simulink model "DC_Motor_PID_Control"  (R2024a)
settings: Solver=VariableStepAuto  StartTime=0.0  StopTime=10.0  RelTol=1e-3
libraries: spsControlledVoltageSourceLib x1, spsCurrentMeasurementLib x1, spsDCMachineLib x1, spsDCVoltageSourceLib x1, slpidlib x1, spspowerguiLib x1
settings Model: Creator=Anjali Sharma  LastModifiedBy=Anjali Sharma

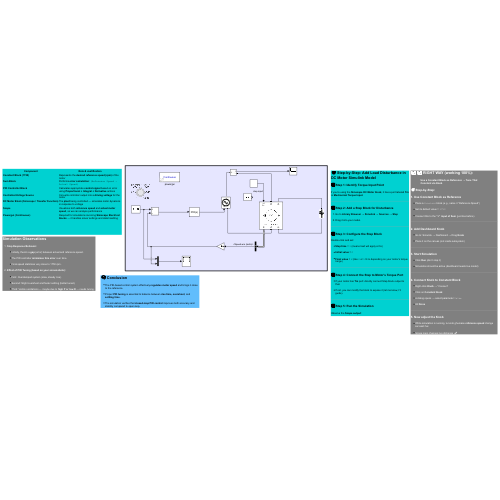
[thumbnail: Simulink's stored preview of the top-level diagram]
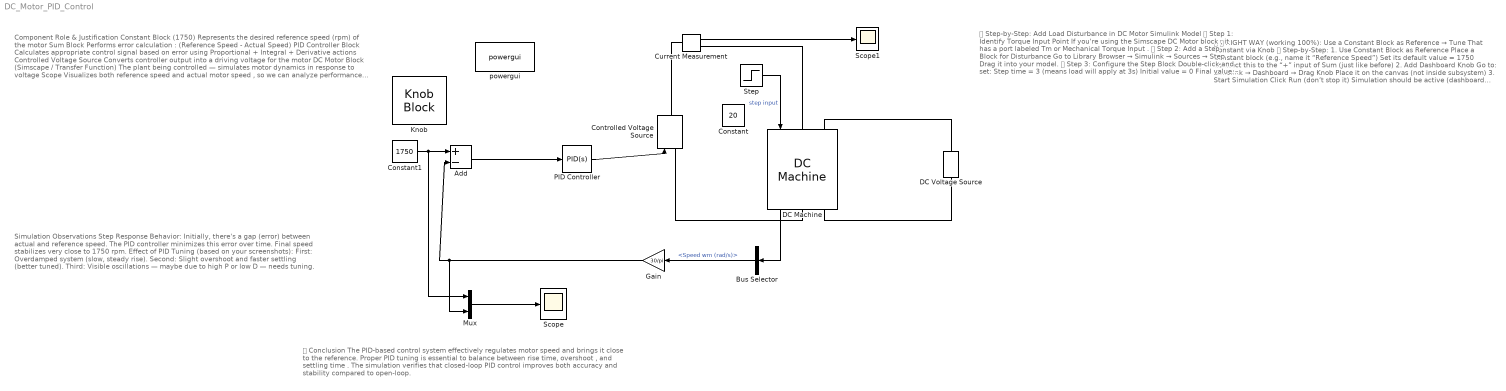
== system DC_Motor_PID_Control ==
  note: ✅ ✅ RIGHT WAY (working 100%):
      | Use a Constant Block as Reference → Tune That Constant via Knob
      | 🧭 Step-by-Step:
      | 1. Use Constant Block as Reference
      | Place a Constant block (e.g., name it “Reference Speed”)
      | Set its default value = 1750
      | Connect this to the “+” input of Sum (just like before)
      | 2. Add Dashboard Knob
      | Go to: Simulink → Dashboard → Drag Knob
      | Place it on the canvas (not inside subsystem)
      | 3. Start Simulation
      | Click Run (don’t stop it)
      | Simulation should be active (dashboard needs live model)
      | 4. Connect Knob to Constant Block
      | Right-click Knob → “Connect”
      | Click on Constant block
      | A dialog opens → select parameter Value
      | Hit Done
      | 5. Now adjust the Knob
      | While simulation is running, tu knob ghumake reference speed change kar sakti hai
      | Scope mein changes live dikhenge 🚀
      | 🧪 Why PID can't directly accept knob:
      | Because the PID input is a dynamic signal , knob can only connect to tunable parameters (like value of Constant or Gain blocks) — not to arbitrary wires or results.
  note: 🧭 Step-by-Step: Add Load Disturbance in DC Motor Simulink Model
      | ✅ Step 1: Identify Torque Input Point
      | If you're using the Simscape DC Motor block , it has a port labeled Tm or Mechanical Torque Input .
      | ✅ Step 2: Add a Step Block for Disturbance
      | Go to Library Browser → Simulink → Sources → Step
      | Drag it into your model.
      | ✅ Step 3: Configure the Step Block
      | Double-click and set:
      | Step time = 3 (means load will apply at 3s)
      | Initial value = 0
      | Final value = X (like 2 or 5 N·m depending on your motor’s torque range)
      | ✅ Step 4: Connect the Step to Motor's Torque Port
      | If your motor has Tm port: directly connect Step block output to that.
      | If not, you can modify the block to expose it (let me know, I’ll guide).
      | ✅ Step 5: Run the Simulation
      | Observe the Scope output :
      | You’ll see a dip in speed at t = 3s due to load.
      | If PID is well-tuned, the motor should recover to 1750 rpm soon after.
      | 🎯 Bonus Tip:
      | Want to test PID strength ? Try:
      | Disturbance = 10 N·m (large)
      | Remove D term from PID → You'll see slower recovery or instability
  note: 🧠 Conclusion
      | The PID-based control system effectively regulates motor speed and brings it close to the reference.
      | Proper PID tuning is essential to balance between rise time, overshoot , and settling time .
      | The simulation verifies that closed-loop PID control improves both accuracy and stability compared to open-loop.
  note: Simulation Observations
      | Step Response Behavior: Initially, there's a gap (error) between actual and reference speed.
      | The PID controller minimizes this error over time.
      | Final speed stabilizes very close to 1750 rpm.
      |
      | Effect of PID Tuning (based on your screenshots): First: Overdamped system (slow, steady rise).
      | Second: Slight overshoot and faster settling (better tuned).
      | Third: Visible oscillations — maybe due to high P or low D — needs tuning.
  note: Component
      | Role & Justification
      |
      | Constant Block (1750)
      | Represents the desired reference speed (rpm) of the motor
      |
      | Sum Block
      | Performs error calculation : (Reference Speed - Actual Speed)
      |
      | PID Controller Block
      | Calculates appropriate control signal based on error using Proportional + Integral + Derivative actions
      |
      | Controlled Voltage Source
      | Converts controller output into a driving voltage for the motor
      |
      | DC Motor Block (Simscape / Transfer Function)
      | The plant being controlled — simulates motor dynamics in response to voltage
      |
      | Scope
      | Visualizes both reference speed and actual motor speed , so we can analyze performance
      |
      | Powergui (Continuous)
      | Required for simulations involving Simscape Electrical blocks — it handles solver settings and data handling
  Add : Sum  Inputs=+-
  Bus Selector : BusSelector  OutputSignals=Speed wm (rad/s)
  Constant : Constant  Value=20
  Constant1 : Constant  Value=1750
  Controlled Voltage Source : spsControlledVoltageSourceLib/Controlled Voltage Source  Initialize=on  Source_Type=AC  Amplitude=0  Phase=0  Frequency=0  Measurements=None
  Current Measurement : spsCurrentMeasurementLib/Current Measurement  PhasorSimulation=off  OutputType=Complex  PSBequivalent=0
  DC Machine : spsDCMachineLib/DC Machine  PresetModel=02: 5HP 240V 1750RPM Field:150V  MechanicalLoad=Torque TL  FieldType=Wound  ShowDetailedParameters=on  MeasurementBus=off  RLa=[0.78 0.016]  RLf=[150 112.5]  Laf=1.234  MachineConstant=Torque constant (N.m/A)  Ke=1.8  Kt=1.8  J=0.05  Bm=0.01  Tf=0  w0=1  Ifinit=1  TsPowergui=0  TsBlock=-1
  DC Voltage Source : spsDCVoltageSourceLib/DC Voltage Source  Amplitude=150  Measurements=None
  Gain : Gain  Gain=30/pi
  Knob : KnobBlock  ScaleMax=3000
  Mux : Mux  Inputs=2
  PID Controller : slpidlib/PID Controller  Controller=PID  Form=Parallel  TimeDomain=Continuous-time  UseExternalTs=off  SampleTime=-1  IntegratorMethod=Forward Euler  FilterMethod=Forward Euler  ControllerParametersSource=internal  P=0.214596036046498  I=5.26646706519129  UseKiTs=off  D=0.00216589040036506  UseExternalDerivativeSource=off  N=5488.43681333471  UseFilter=on  TunerSelectOption=Transfer Function Based (PID Tuner App)  InitialConditionSource=internal  InitialConditionForIntegrator=0  InitialConditionForFilter=0  DifferentiatorICPrevScaledInput=0  ExternalReset=none  TrackingMode=off  Kt=1  LimitOutput=off  SatLimitsSource=internal  UpperSaturationLimit=inf  LowerSaturationLimit=-inf  LinearizeAsGain=on  AntiWindupMode=none  Kb=1  LimitIntegrator=off  UpperIntegratorSaturationLimit=inf  LowerIntegratorSaturationLimit=-inf  POutMin=[]  POutMax=[]  IOutMin=[]  IOutMax=[]  DOutMin=[]  DOutMax=[]  NOutMin=[]  NOutMax=[]  SumOutMin=[]  SumOutMax=[]  SaturationOutMin=[]  SaturationOutMax=[]  PParamMin=[]  PParamMax=[]  IParamMin=[]  IParamMax=[]  DParamMin=[]  DParamMax=[]  NParamMin=[]  NParamMax=[]  KbParamMin=[]  KbParamMax=[]  KtParamMin=[]  KtParamMax=[]  KbOutMin=[]  KbOutMax=[]  KtOutMin=[]  KtOutMax=[]  IntegratorOutMin=[]  IntegratorOutMax=[]  FilterOutMin=[]  FilterOutMax=[]  SumI1OutMin=[]  SumI1OutMax=[]  SumI2OutMin=[]  SumI2OutMax=[]  SumI3OutMin=[]  SumI3OutMax=[]  SumI4OutMin=[]  SumI4OutMax=[]  SumDOutMin=[]  SumDOutMax=[]  DifferentiatorOutMin=[]  DifferentiatorOutMax=[]  FilterDiffOutCoefMin=[]  FilterDiffOutCoefMax=[]  ReciprocalOutMin=[]  ReciprocalOutMax=[]  SumDenOutMin=[]  SumDenOutMax=[]  SumNumOutMin=[]  SumNumOutMax=[]  DivideOutMin=[]  DivideOutMax=[]  UdiffTsProdOutMin=[]  UdiffTsProdOutMax=[]  NTsProdOutMin=[]  NTsProdOutMax=[]  UintegralTsProdOutMin=[]  UintegralTsProdOutMax=[]  UngainTsProdOutMin=[]  UngainTsProdOutMax=[]  ClampingZeroOutDataTypeStr=Inherit: Inherit via back propagation  ClampingZeroOutMin=[]  ClampingZeroOutMax=[]  FilterDenConstantOutDataTypeStr=Inherit: Inherit via back propagation  FilterDenConstantOutMin=[]  FilterDenConstantOutMax=[]  PCopyOutDataTypeStr=Inherit: Inherit via back propagation  PCopyOutMin=[]  PCopyOutMax=[]  NCopyOutDataTypeStr=Inherit: Inherit via back propagation  NCopyOutMin=[]  NCopyOutMax=[]  IntegratorContinuousStateAttributes=''  IntegratorStateMustResolveToSignalObject=off  IntegratorRTWStateStorageClass=Auto  FilterContinuousStateAttributes=''  FilterStateMustResolveToSignalObject=off  FilterRTWStateStorageClass=Auto  ParallelPVariant=InternalParameters  IdealPVariant=Disabled  IVariant=InternalParameters  DVariant=InternalParameters  IntegratorVariant=Continuous  SatVariant=Disabled  AWVariant=Passthrough  PCopyVariant=Disabled  TRVariant=Disabled  FdbkBlocksVariant=Forward  IdealPFdbkVariant=Disabled  SatFdbkVariant=Disabled  DerivativeFilterVariant=ContFilter  NVariant=InternalParameters  NCopyVariant=Disabled  FilterICVariant=InternalICsFilter  IntegratorICVariant=InternalICs  ExternalResetVariant=Disabled  TRSumVariant=Passthrough  SumFdbkVariant=Disabled  SumVariant=Sum_PID  TsampFilterVariant=InternalTs  TsampNgainVariant=Passthrough  TsampIntegralVariant=Disabled_SignalSpec  ExternalSaturationOutDataTypeStr=Inherit: Same as second input  DerivativeSourceVariant=ErrorSignal
  Scope : Scope
  Scope1 : Scope
  Step : Step  Time=3  After=2  SampleTime=0
  powergui : spspowerguiLib/powergui  Priority=1  SimulationMode=Continuous  SampleTime=50e-6  frequency=60  Iterations=50  frequencyindice=0  Pbase=100e6  ErrMax=1e-4  UnitsV=kV  UnitsW=MW  buscounter=0  FunctionMessages=off  echomessages=off  EnableUseOfTLC=off  CurrentSourceSwitches=off  DisableSnubberDevices=off  DisableRonSwitches=off  DisableVfSwitches=off  DisplayEquations=off  AutomaticDiscreteSolvers=off  SolverType=Tustin/Backward Euler (TBE)  Interpol=off  ExternalGateDelay=off  methode=off  Ts=100  x0status=blocks  SPID=on  SwTol=0  HookPort=off  NonlinearTolerance=1e-4  nMaxIteration=100  ContinueOnMaxIteration=off  RestoreLinks=warning  ResistiveCurrentMeasurement=off  Frange=[0:2:500]  Ylog=off  Xlog=on  ShowGrid=off  save=off  variable=ZData  structure=0  ZoomFFT=off  StartTime=0.0  cycles=1  DisplayStyle=1  fundamental=60  FreqAxis=off  MaxFrequency=1000  frequencyindicesteady=1  RmsSteady=1  display=off
  wires:
  PID Controller/1 -> Controlled Voltage Source/1
  DC Machine/1 -> Bus Selector/1
  Bus Selector/1 -> Gain/1  "<Speed wm (rad/s)>"
  Gain/1 -> Mux/2, Add/2
  Add/1 -> PID Controller/1
  Mux/1 -> Scope/1
  Current Measurement/1 -> Scope1/1
  Step/1 -> DC Machine/1  "step input"
  Constant1/1 -> Mux/1, Add/1
  connections:
  DC Voltage Source/RConn1 -- DC Machine/LConn2
  DC Voltage Source/LConn1 -- DC Machine/RConn2
  Controlled Voltage Source/LConn1 -- DC Machine/RConn1
  Current Measurement/LConn1 -- Controlled Voltage Source/RConn1
  Current Measurement/RConn1 -- DC Machine/LConn1
